simulink model "model_simulink"  (R2022a)
settings: Solver=ode1  StartTime=0.0  StopTime=10  FixedStep=0.01  RelTol=1e-3
values from neighbouring files (symbols this model uses):
  A = [-0.0110  0.0433  1.7295  -7.1876 ... (first row only)    [model0001.m]
  B = [-0.4412 ... (first row only)    [model0001.m]
  C = eye(4)    [model0001.m]
  D = [0;0;0;0]    [model0001.m]
undefined symbols (not defined in the file or in its folder): deg, rad, s
libraries: simulink_extras x2, aerolibconvert2 x1, cstblocks x1, slpidlib x1
settings Model: Creator=root  LastModifiedBy=aleksejpasenko
settings SolverCC: AlgebraicLoopSolver=TrustRegion
settings DataIOCC: ReturnWorkspaceOutputs=off
settings DebuggingCC: UnconnectedInputMsg=warning  UnconnectedOutputMsg=warning  UnconnectedLineMsg=warning  SFMachineParentedDataDiag=warning

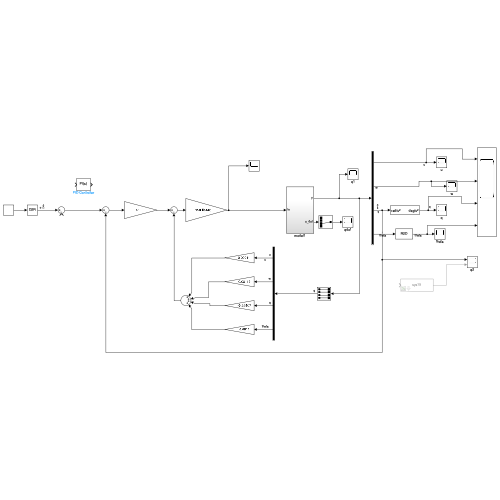
[thumbnail: Simulink's stored preview of the top-level diagram]
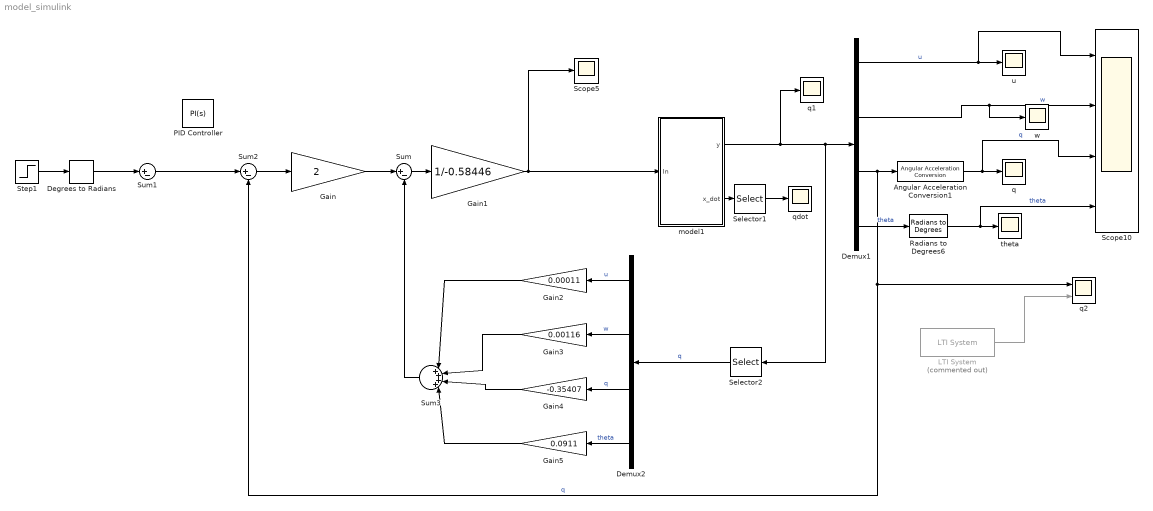
== system model_simulink ==
  Angular Acceleration Conversion1 : aerolibconvert2/Angular Acceleration Conversion  IU=rad/s^2  OU=deg/s^2
      settings: SourceProductBaseCode=AE
  Degrees to Radians : simulink_extras/Transformations/Degrees to Radians
  Demux1 : Demux
  Demux2 : Demux
  Gain : Gain  Gain=2
  Gain1 : Gain  Gain=1/-0.58446
  Gain2 : Gain  Gain=0.00011
  Gain3 : Gain  Gain=0.00116
  Gain4 : Gain  Gain=-0.35407
  Gain5 : Gain  Gain=0.0911
  LTI System : cstblocks/LTI System  Commented=on  sys=sys15  IC=[]
  PID Controller : slpidlib/PID Controller  Controller=PI  Form=Parallel  TimeDomain=Continuous-time  UseExternalTs=off  SampleTime=-1  IntegratorMethod=Forward Euler  FilterMethod=Forward Euler  ControllerParametersSource=internal  P=2  I=5  UseKiTs=off  D=0  N=100  UseFilter=on  TunerSelectOption=Transfer Function Based (PID Tuner App)  InitialConditionSource=internal  InitialConditionForIntegrator=0  InitialConditionForFilter=0  DifferentiatorICPrevScaledInput=0  ExternalReset=none  TrackingMode=off  Kt=1  LimitOutput=off  SatLimitsSource=internal  UpperSaturationLimit=inf  LowerSaturationLimit=-inf  LinearizeAsGain=on  AntiWindupMode=none  Kb=1  POutMin=[]  POutMax=[]  IOutMin=[]  IOutMax=[]  DOutMin=[]  DOutMax=[]  NOutMin=[]  NOutMax=[]  SumOutMin=[]  SumOutMax=[]  SaturationOutMin=[]  SaturationOutMax=[]  PParamMin=[]  PParamMax=[]  IParamMin=[]  IParamMax=[]  DParamMin=[]  DParamMax=[]  NParamMin=[]  NParamMax=[]  KbParamMin=[]  KbParamMax=[]  KtParamMin=[]  KtParamMax=[]  KbOutMin=[]  KbOutMax=[]  KtOutMin=[]  KtOutMax=[]  IntegratorOutMin=[]  IntegratorOutMax=[]  FilterOutMin=[]  FilterOutMax=[]  SumI1OutMin=[]  SumI1OutMax=[]  SumI2OutMin=[]  SumI2OutMax=[]  SumI3OutMin=[]  SumI3OutMax=[]  SumI4OutMin=[]  SumI4OutMax=[]  SumDOutMin=[]  SumDOutMax=[]  DifferentiatorOutMin=[]  DifferentiatorOutMax=[]  FilterDiffOutCoefMin=[]  FilterDiffOutCoefMax=[]  ReciprocalOutMin=[]  ReciprocalOutMax=[]  SumDenOutMin=[]  SumDenOutMax=[]  SumNumOutMin=[]  SumNumOutMax=[]  DivideOutMin=[]  DivideOutMax=[]  UdiffTsProdOutMin=[]  UdiffTsProdOutMax=[]  NTsProdOutMin=[]  NTsProdOutMax=[]  UintegralTsProdOutMin=[]  UintegralTsProdOutMax=[]  UngainTsProdOutMin=[]  UngainTsProdOutMax=[]  IntegratorContinuousStateAttributes=''  IntegratorStateMustResolveToSignalObject=off  IntegratorRTWStateStorageClass=Auto  FilterContinuousStateAttributes=''  FilterStateMustResolveToSignalObject=off  FilterRTWStateStorageClass=Auto  ParallelPVariant=InternalParameters  IdealPVariant=Disabled  IVariant=InternalParameters  DVariant=Disabled  IntegratorVariant=Continuous  SatVariant=Disabled  AWVariant=Passthrough  PCopyVariant=Disabled  TRVariant=Disabled  FdbkBlocksVariant=Forward  IdealPFdbkVariant=Disabled  SatFdbkVariant=Disabled  DerivativeFilterVariant=Disabled  NVariant=Disabled  NCopyVariant=Disabled_SignalSpec  FilterICVariant=Disabled  IntegratorICVariant=InternalICs  ExternalResetVariant=Disabled  TRSumVariant=Passthrough  SumFdbkVariant=Disabled  SumVariant=Sum_PI  TsampFilterVariant=InternalTs  TsampNgainVariant=Passthrough  TsampIntegralVariant=Passthrough  ExternalSaturationOutDataTypeStr=Inherit: Same as second input  aMode=0
  Radians to Degrees6 : simulink_extras/Transformations/Radians to Degrees
  Scope10 : Scope  NumInputPorts=4
  Scope5 : Scope
  Selector1 : Selector  InputPortWidth=4  IndexOptions=Index vector (dialog)  Indices=3  OutputSizes=1
  Selector2 : Selector  InputPortWidth=4  IndexOptions=Index vector (dialog)  Indices=[1 2 3 4]  OutputSizes=1
  Step1 : Step  Time=0  After=-1  SampleTime=0
  Sum : Sum  Inputs=|+-
  Sum1 : Sum  Inputs=|+-
  Sum2 : Sum  Inputs=|+-
  Sum3 : Sum  Inputs=|++++|
  model1 : Subsystem
  q : Scope
  q1 : Scope
  q2 : Scope  NumInputPorts=2
  qdot : Scope
  theta : Scope
  u : Scope
  w : Scope
  wires:
  Demux1/2 -> w/1, Scope10/2  "w"
  Radians to Degrees6/1 -> theta/1, Scope10/4  "theta"
  Demux2/3 -> Gain4/1  "q"
  Gain2/1 -> Sum3/1
  Demux2/1 -> Gain2/1  "u"
  Gain4/1 -> Sum3/3
  model1/2(x_dot) -> Selector1/1
  Selector2/1 -> Demux2/1  "q"
  Gain1/1 -> model1/1(In), Scope5/1
  Gain5/1 -> Sum3/4
  Gain3/1 -> Sum3/2
  Demux2/4 -> Gain5/1  "theta"
  Step1/1 -> Degrees to Radians/1
  Demux1/1 -> Scope10/1, u/1  "u"
  Sum2/1 -> Gain/1
  model1/1(y) -> q1/1, Selector2/1, Demux1/1
  Sum3/1 -> Sum/2
  Demux2/2 -> Gain3/1  "w"
  Sum/1 -> Gain1/1
  Selector1/1 -> qdot/1
  Demux1/3 -> Angular Acceleration Conversion1/1, Sum2/2, q2/1  "q"
  Demux1/4 -> Radians to Degrees6/1  "theta"
  Gain/1 -> Sum/1
  Degrees to Radians/1 -> Sum1/1
  Angular Acceleration Conversion1/1 -> Scope10/3, q/1  "q"
  LTI System/1 -> q2/2
  Sum1/1 -> Sum2/1

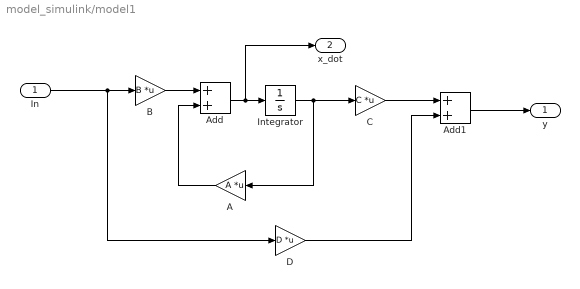
== system model_simulink/model1 ==
  In : Inport
  A : Gain  Gain=A  Multiplication=Matrix(K*u)
  Add : Sum
  Add1 : Sum
  B : Gain  Gain=B  Multiplication=Matrix(K*u)
  C : Gain  Gain=C  Multiplication=Matrix(K*u)
  D : Gain  Gain=D  Multiplication=Matrix(K*u)
  Integrator : Integrator
  y : Outport  VectorParamsAs1DForOutWhenUnconnected=off
  x_dot : Outport  Port=2
  wires:
  B/1 -> Add/1
  Integrator/1 -> A/1, C/1
  Add/1 -> x_dot/1, Integrator/1
  C/1 -> Add1/1
  In/1 -> B/1, D/1
  D/1 -> Add1/2
  A/1 -> Add/2
  Add1/1 -> y/1
